simulink model "MPU9250_Simulink_Arduino"  (R2020a)
settings: Solver=FixedStepDiscrete  StartTime=0.0  StopTime=inf  FixedStep=0.001  RelTol=1e-3  EnableMultiTasking=on
libraries: arduinolib x5
settings Model: SILPILModeSetting=veronly  EnablePacing=on  ExtModeTrigDuration=2  Creator=rodri  LastModifiedBy=rodri
settings OptimizationCC: EnhancedBackFolding=on  PassReuseOutputArgsAs=Individual arguments  ZeroExternalMemoryAtStartup=off  ZeroInternalMemoryAtStartup=off  MaxStackSize=64  OptimizeBlockOrder=speed  DifferentSizesBufferReuse=on  OptimizationCustomize=off  EfficientTunableParamExpr=on
settings DebuggingCC: ParameterTunabilityLossMsg=error
settings HardwareCC: ProdBitPerInt=16  ProdBitPerPointer=16  ProdBitPerSizeT=16  ProdBitPerPtrDiffT=16  ProdLargestAtomicFloat=None  ProdWordSize=8  ProdHWDeviceType=Atmel->AVR
settings SFSimCC: MATLABDynamicMemAlloc=off
settings RTWCC: SystemTargetFile=ert.tlc  HardwareBoard=Arduino Mega 2560  TLCOptions=-aInlineSetEventsForThisBaseRateFcn=TLC_FALSE -aSuppressMultiTaskScheduler=TLC_FALSE -aRateBasedStepFcn=1  TemplateMakefile=ert_default_tmf  Toolchain=Arduino AVR  BuildConfiguration=Faster Runs
settings CodeAppCC: ForceParamTrailComments=on  IgnoreCustomStorageClasses=off  OperatorAnnotations=on  SimulinkDataObjDesc=on  SFDataObjDesc=on  InsertBlockDesc=on
settings ERTTargetCC: SupportContinuousTime=on  SupportVariableSizeSignals=on  ExtModeStaticAllocSize=2048

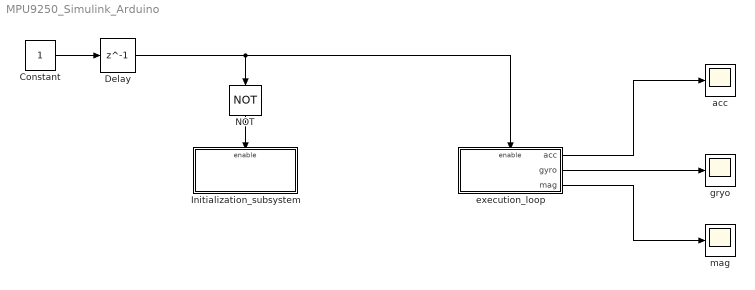
== system MPU9250_Simulink_Arduino ==
  Constant : Constant
  Delay : Delay  DelayLength=1
  Initialization_subsystem : Subsystem  TreatAsAtomicUnit=on
  NOT : Logic  Operator=NOT  AllPortsSameDT=off  OutDataTypeStr=boolean
  acc : Scope
  execution_loop : Subsystem  TreatAsAtomicUnit=on
  gryo : Scope
  mag : Scope
  wires:
  Constant/1 -> Delay/1
  Delay/1 -> execution_loop/Enable, NOT/1
  execution_loop/1(acc) -> acc/1
  execution_loop/2(gyro) -> gryo/1
  execution_loop/3(mag) -> mag/1
  NOT/1 -> Initialization_subsystem/Enable

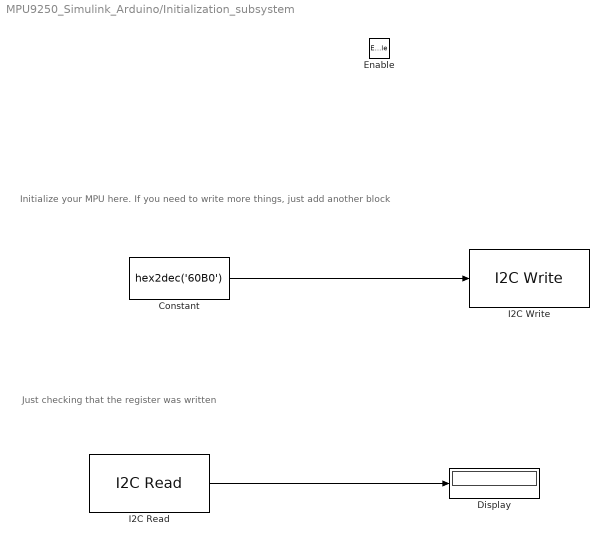
== system MPU9250_Simulink_Arduino/Initialization_subsystem ==
  note: Just checking that the register was written
  note: Initialize your MPU here. If you need to write more things, just add another block
  Enable : EnablePort
  Constant : Constant  Value=hex2dec('60B0')  OutDataTypeStr=uint16
  Display : Display
  I2C Read : arduinolib/I2C Read  I2CModule=0  Mode=Master  SlaveAddress=10  SlaveByteOrder=BigEndian  Direction=Receiver  RegisterAddressMode=on  RegisterAddress=0  SlaveDataType=uint8  DataLength=1  NoAck=off  RepeatedStart=off  OutputStatus=off  blockPlatform=ARDUINO  SampleTime=0.1
      settings: SourceProductBaseCode=ARDUINO
  I2C Write : arduinolib/I2C Write  I2CModule=0  Mode=Master  SlaveAddress=10  SlaveByteOrder=BigEndian  Direction=Transmitter  RegisterAddressMode=on  RegisterAddress=0  SlaveDataType=uint8  DataLength=1  NoAck=off  RepeatedStart=off  OutputStatus=off  blockPlatform=ARDUINO
      settings: SourceProductBaseCode=ARDUINO
  wires:
  Constant/1 -> I2C Write/1
  I2C Read/1 -> Display/1

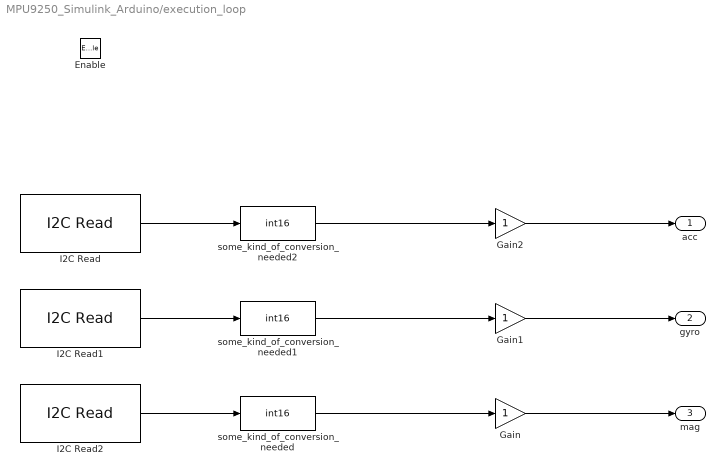
== system MPU9250_Simulink_Arduino/execution_loop ==
  Enable : EnablePort
  Gain : Gain
  Gain1 : Gain
  Gain2 : Gain
  I2C Read : arduinolib/I2C Read  I2CModule=0  Mode=Master  SlaveAddress=10  SlaveByteOrder=BigEndian  Direction=Receiver  RegisterAddressMode=on  RegisterAddress=0  SlaveDataType=uint8  DataLength=1  NoAck=off  RepeatedStart=off  OutputStatus=off  blockPlatform=ARDUINO  SampleTime=0.1
      settings: SourceProductBaseCode=ARDUINO
  I2C Read1 : arduinolib/I2C Read  I2CModule=0  Mode=Master  SlaveAddress=10  SlaveByteOrder=BigEndian  Direction=Receiver  RegisterAddressMode=on  RegisterAddress=0  SlaveDataType=uint8  DataLength=1  NoAck=off  RepeatedStart=off  OutputStatus=off  blockPlatform=ARDUINO  SampleTime=0.1
      settings: SourceProductBaseCode=ARDUINO
  I2C Read2 : arduinolib/I2C Read  I2CModule=0  Mode=Master  SlaveAddress=10  SlaveByteOrder=BigEndian  Direction=Receiver  RegisterAddressMode=on  RegisterAddress=0  SlaveDataType=uint8  DataLength=1  NoAck=off  RepeatedStart=off  OutputStatus=off  blockPlatform=ARDUINO  SampleTime=0.1
      settings: SourceProductBaseCode=ARDUINO
  some_kind_of_conversion_needed : DataTypeConversion  OutDataTypeStr=int16  ConvertRealWorld=Stored Integer (SI)
  some_kind_of_conversion_needed1 : DataTypeConversion  OutDataTypeStr=int16  ConvertRealWorld=Stored Integer (SI)
  some_kind_of_conversion_needed2 : DataTypeConversion  OutDataTypeStr=int16  ConvertRealWorld=Stored Integer (SI)
  acc : Outport
  gyro : Outport  Port=2
  mag : Outport  Port=3
  wires:
  I2C Read2/1 -> some_kind_of_conversion_needed/1
  I2C Read1/1 -> some_kind_of_conversion_needed1/1
  I2C Read/1 -> some_kind_of_conversion_needed2/1
  some_kind_of_conversion_needed/1 -> Gain/1
  Gain/1 -> mag/1
  some_kind_of_conversion_needed1/1 -> Gain1/1
  Gain1/1 -> gyro/1
  some_kind_of_conversion_needed2/1 -> Gain2/1
  Gain2/1 -> acc/1
